simulink model "LinearRLC1Model"  (R2014a)
settings: Solver=ode4  StartTime=0.0  StopTime=5  FixedStep=0.1  RelTol=1e-3
settings Model: Creator=SH343  LastModifiedBy=SH343
settings DataIOCC: SignalLoggingSaveFormat=ModelDataLogs
settings DebuggingCC: MultiTaskDSMMsg=warning  MultiTaskCondExecSysMsg=none
settings RTWCC: IncludeERTFirstTime=on

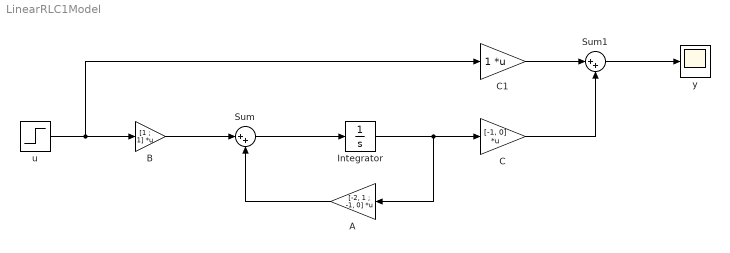
== system LinearRLC1Model ==
  A : Gain  Gain=[-2, 1 ; -1, 0]  Multiplication=Matrix(K*u)
  B : Gain  Gain=[1 ; 1]  Multiplication=Matrix(K*u)
  C : Gain  Gain=[-1, 0]  Multiplication=Matrix(K*u)
  C1 : Gain  Multiplication=Matrix(K*u)
  Integrator : Integrator
  Sum : Sum  Inputs=|++
  Sum1 : Sum  Inputs=|++
  u : Step  Time=0  SampleTime=0
  y : Scope
  wires:
  u/1 -> C1/1, B/1
  Integrator/1 -> A/1, C/1
  Sum/1 -> Integrator/1
  A/1 -> Sum/2
  B/1 -> Sum/1
  Sum1/1 -> y/1
  C/1 -> Sum1/2
  C1/1 -> Sum1/1
